simulink model "UpperLimb_Controller"  (R2024b)
settings: Solver=VariableStepAuto  StartTime=0.0  StopTime=10.0  RelTol=1e-3
settings Model: Creator=jakub  LastModifiedBy=jakub

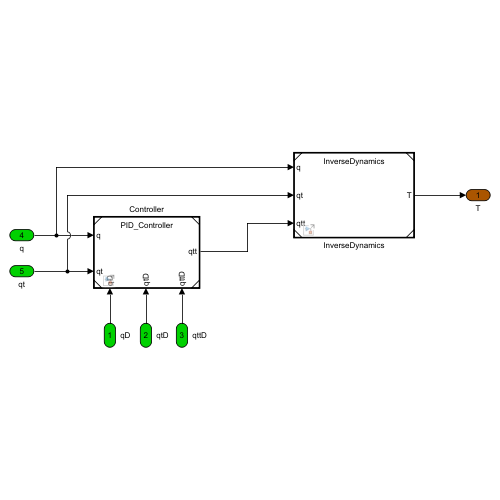
[thumbnail: Simulink's stored preview of the top-level diagram]
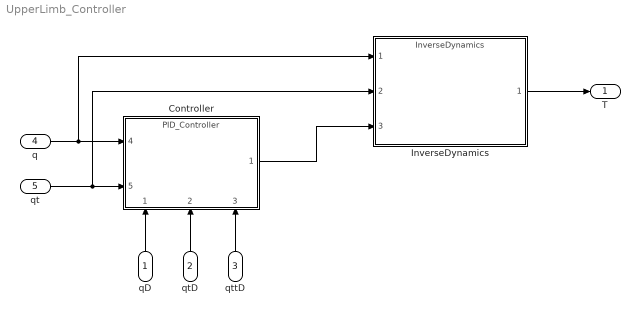
== system UpperLimb_Controller ==
  qD : Inport  OutDataTypeStr=double  Unit=rad  PortDimensions=[2 1]  SampleTime=0
  qtD : Inport  Port=2  OutDataTypeStr=double  Unit=rad/s  PortDimensions=[2 1]  SampleTime=0
  qttD : Inport  Port=3  OutDataTypeStr=double  Unit=rad/s^2  PortDimensions=[2 1]  SampleTime=0
  q : Inport  Port=4  OutDataTypeStr=double  Unit=rad  PortDimensions=[2 1]  SampleTime=0
  qt : Inport  Port=5  OutDataTypeStr=double  Unit=rad/s  PortDimensions=[2 1]  SampleTime=0
  Controller : ModelReference  ModelNameDialog=PID_Controller.slx  SimulationMode=Normal  ModelReferenceVersion=1.5
      settings: PortSchema="{\"entries\":[{\"content\":{\"sides\":[{\"content\":{\"connectorIds\":[\"In4\",\"In5\"]},\"type\":\"ConnectorPlacement.EquallySpacedRectSide\",\"uuid\":\"5cad86c4-3157-45b7-b98d-461c1671640b\"},{\"content\":{\"connectorIds\":[\"Out1\"],\"side\":\"RIGHT\"},\"type\":\"ConnectorPlacement.EquallySpacedRectSide\",\"uuid\":\"d045131f-e11b-44ce-af03-04833f64aa0e\"},{\"content\":{\"side\":\"TOP\"},\"type\":\"ConnectorPlacement.EquallySpacedRectSide\",\"uuid\":\"4be6d916-921b-45bd-b706-86e8993c7e38\"},{\"content\":{\"connectorIds\":[\"In1\",\"In2\",\"In3\"],\"side\":\"BOTTOM\"},\"type\":\"ConnectorPlacement.EquallySpacedRectSide\",\"uuid\":\"1a480b1d-7167-4366-b766-33e2dc0e3215\"}]},\"type\":\"ConnectorPlacement.EquallySpacedConnector\",\"uuid\":\"82bf8fe4-c499-45da-b9c3-9b2a123cd3ef\"}],\"packageUris\":[\"http://schema.mathworks.com/mf0/Connector/R2020b\"],\"version\":\"1.0\"}"
  InverseDynamics : ModelReference  ModelNameDialog=InverseDynamics.slx  SimulationMode=Normal  ModelReferenceVersion=1.3
  T : Outport  OutDataTypeStr=double  Unit=N*m  PortDimensions=[2 1]  SampleTime=0
  wires:
  Controller/1 -> InverseDynamics/3
  qttD/1 -> Controller/3
  qtD/1 -> Controller/2
  qt/1 -> InverseDynamics/2, Controller/5
  q/1 -> Controller/4, InverseDynamics/1
  qD/1 -> Controller/1
  InverseDynamics/1 -> T/1
